simulink model "unicycle"  (R2025b)
settings: Solver=ode5  StartTime=0.0  StopTime=40  FixedStep=1e-3  MaxStep=0.01  RelTol=1e-3
libraries: dspsigops x1
settings Model: Creator=Cris  LastModifiedBy=Cris
settings DebuggingCC: UnderspecifiedInitializationDetection=Classic  MergeDetectMultiDrivingBlocksExec=none
settings ModelReferenceCC: PropagateSignalLabelsOutOfModel=off

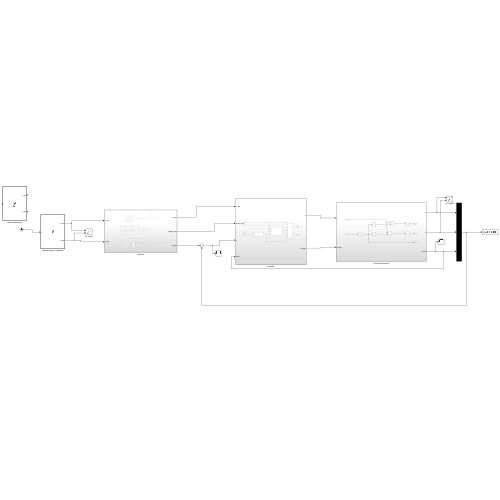
[thumbnail: Simulink's stored preview of the top-level diagram]
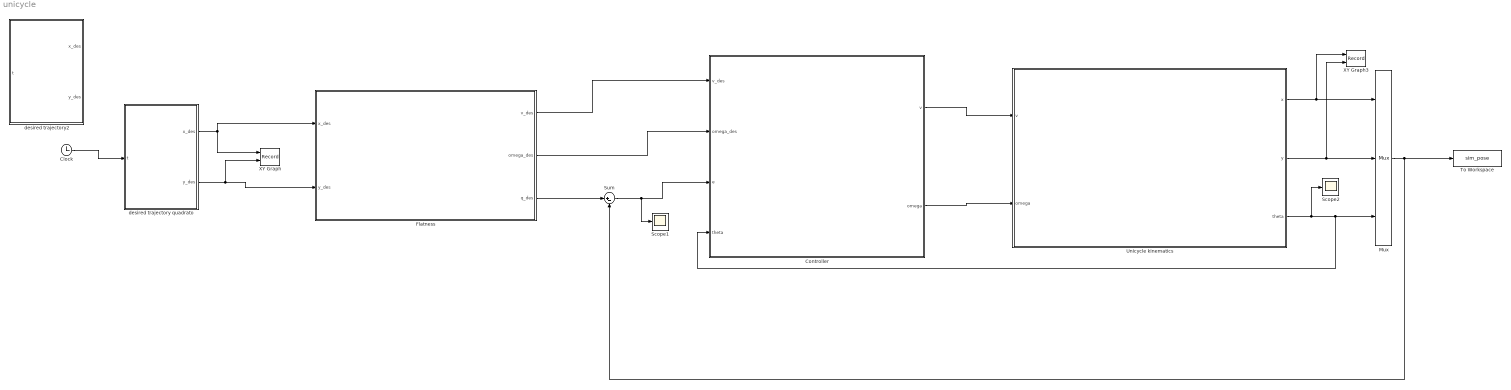
== system unicycle ==
  Clock : Clock
  Controller : Subsystem
  Flatness : Subsystem
  Mux : Mux  Inputs=3
  Scope1 : Scope
      settings: ActiveDisplayYMinimum=-1  ActiveDisplayYMaximum=1  DataLoggingVariableName=ScopeData3  DataLoggingSaveFormat=Array
  Scope2 : Scope
      settings: ActiveDisplayYMinimum=-1.1717356950439886  ActiveDisplayYMaximum=10.422944252013369  DataLoggingSaveFormat=Array
  Sum : Sum  Inputs=|+-
  To Workspace : ToWorkspace  VariableName=sim_pose  SaveFormat=Timeseries  SampleTime=-1
  Unicycle kinematics : Subsystem
  XY Graph : Record  NumPorts=2.0  FileSettingsInternal="{\"entries\":[{\"content\":{\"excelSettings\":{\"content\":{},\"type\":\"Streamout.ExcelSettings\"},\"parquetSettings\":{\"content\":{},\"type\":\"Streamout.ParquetSettings\"}},\"type\":\"Streamout.FileSettingStorage\",\"uuid\":\"\"}],\"packageUris\":[\"http:\\/\\/schema.mathworks.com\\/mf0\\/streamout_blocks\\/R2020a\"],\"version\":\"1.0\"}"  FrameSettings=[0, 0]  Layout=[1 1]  SignalsInternal="{\"entries\":[{\"content\":{\"signals\":[{\"content\":{\"blockPath\":[],\"dimensions\":[1],\"domain\":\"\",\"lineColor\":\"#a2142f\",\"plots\":[ 1 ],\"port\":1,\"sid\":[\"\"],\"signalID\":1,\"signalName\":\"desired trajectory quadrato:1\"},\"type\":\"RecordBlkView.Signal\",\"uuid\":\"\"},{\"content\":{\"blockPath\":[],\"dimensions\":[1],\"domain\":\"\",\"lineColor\":\"#139fff\",\"plots\":[ 1 ],\"port\":2,\"sid\":[\"\"],\"signalID\":2,\"signalName\":\"desired trajectory quadrato:2\"},\"type\":\"RecordBlkView.Signal\",\"uuid\":\"\"}]},\"type\":\"RecordBlkView.InputSignals\",\"uuid\":\"\"}],\"packageUris\":[\"http:\\/\\/schema.mathworks.com\\/mf0\\/streamout_blocks\\/R2020a\"],\"version\":\"1.0\"}"  VisualizationBindings="{\"xyplotplugin\":{\"info\":[{\"series\":[{\"bindingParametersList\":[{\"parameter\":\"X-Axis\",\"signalID\":1,\"signalName\":\"desired trajectory quadrato:1\"},{\"parameter\":\"Y-Axis\",\"signalID\":2,\"signalName\":\"desired trajectory quadrato:2\"}],\"seriesID\":0}],\"subplotID\":1}]}}"  CompatibilityTag=XY
  XY Graph3 : Record  NumPorts=2.0  FileSettingsInternal="{\"entries\":[{\"content\":{\"excelSettings\":{\"content\":{},\"type\":\"Streamout.ExcelSettings\"},\"parquetSettings\":{\"content\":{},\"type\":\"Streamout.ParquetSettings\"}},\"type\":\"Streamout.FileSettingStorage\",\"uuid\":\"\"}],\"packageUris\":[\"http:\\/\\/schema.mathworks.com\\/mf0\\/streamout_blocks\\/R2020a\"],\"version\":\"1.0\"}"  FrameSettings=[0, 0]  Layout=[1 1]  SignalsInternal="{\"entries\":[{\"content\":{\"signals\":[{\"content\":{\"blockPath\":[],\"dimensions\":[1],\"domain\":\"\",\"lineColor\":\"#a2142f\",\"plots\":[ 1 ],\"port\":1,\"sid\":[\"\"],\"signalID\":1,\"signalName\":\"Unicycle kinematics:1\"},\"type\":\"RecordBlkView.Signal\",\"uuid\":\"\"},{\"content\":{\"blockPath\":[],\"dimensions\":[1],\"domain\":\"\",\"lineColor\":\"#139fff\",\"plots\":[ 1 ],\"port\":2,\"sid\":[\"\"],\"signalID\":2,\"signalName\":\"Unicycle kinematics:2\"},\"type\":\"RecordBlkView.Signal\",\"uuid\":\"\"}]},\"type\":\"RecordBlkView.InputSignals\",\"uuid\":\"\"}],\"packageUris\":[\"http:\\/\\/schema.mathworks.com\\/mf0\\/streamout_blocks\\/R2020a\"],\"version\":\"1.0\"}"  VisualizationBindings="{\"xyplotplugin\":{\"info\":[{\"series\":[{\"bindingParametersList\":[{\"parameter\":\"X-Axis\",\"signalID\":1,\"signalName\":\"Unicycle kinematics:1\"},{\"parameter\":\"Y-Axis\",\"signalID\":2,\"signalName\":\"Unicycle kinematics:2\"}],\"seriesID\":0}],\"subplotID\":1}]}}"  CompatibilityTag=XY
  desired trajectory quadrato : MATLAB Function  TreatAsAtomicUnit=on
  desired trajectory2 : MATLAB Function  TreatAsAtomicUnit=on
  wires:
  Flatness/1(v_des) -> Controller/1(v_des)
  Flatness/2(omega_des) -> Controller/2(omega_des)
  Flatness/3(q_des) -> Sum/1
  Sum/1 -> Scope1/1, Controller/3(e)
  Unicycle kinematics/1(x) -> XY Graph3/1, Mux/1
  Unicycle kinematics/2(y) -> XY Graph3/2, Mux/2
  Unicycle kinematics/3(theta) -> Scope2/1, Controller/4(theta), Mux/3
  Mux/1 -> To Workspace/1, Sum/2
  Controller/2(omega) -> Unicycle kinematics/2(omega)
  Controller/1(v) -> Unicycle kinematics/1(v)
  desired trajectory quadrato/1(x_des) -> Flatness/1(x_des), XY Graph/1
  desired trajectory quadrato/2(y_des) -> Flatness/2(y_des), XY Graph/2
  Clock/1 -> desired trajectory quadrato/1(t)

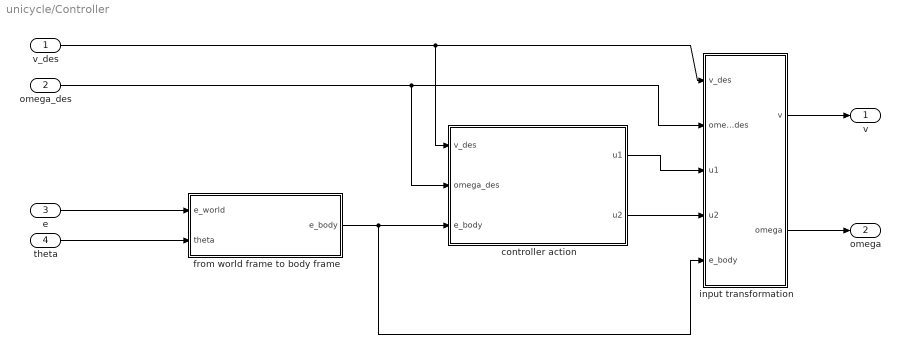
== system unicycle/Controller ==
  v_des : Inport
  omega_des : Inport  Port=2
  e : Inport  Port=3
  theta : Inport  Port=4
  controller action : MATLAB Function  TreatAsAtomicUnit=on
  from world frame to body frame : MATLAB Function  TreatAsAtomicUnit=on
  input transformation : MATLAB Function  TreatAsAtomicUnit=on
  v : Outport
  omega : Outport  Port=2
  wires:
  e/1 -> from world frame to body frame/1(e_world)
  theta/1 -> from world frame to body frame/2(theta)
  from world frame to body frame/1(e_body) -> input transformation/5(e_body), controller action/3(e_body)
  v_des/1 -> controller action/1(v_des), input transformation/1(v_des)
  controller action/2(u2) -> input transformation/4(u2)
  input transformation/2(omega) -> omega/1
  input transformation/1(v) -> v/1
  omega_des/1 -> input transformation/2(omega_des), controller action/2(omega_des)
  controller action/1(u1) -> input transformation/3(u1)

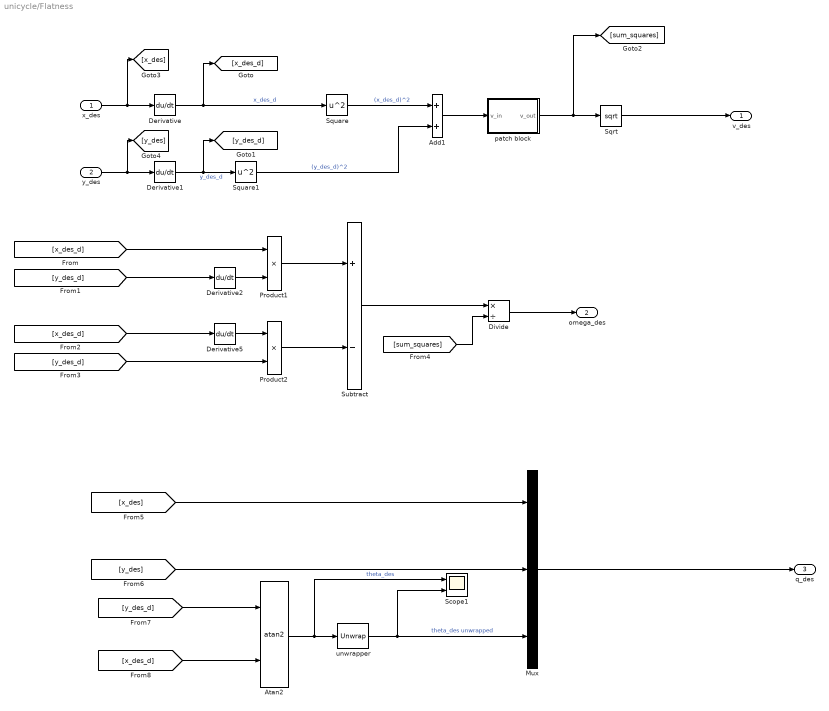
== system unicycle/Flatness ==
  x_des : Inport
  y_des : Inport  Port=2
  Add1 : Sum
  Atan2 : Trigonometry  Operator=atan2
  Derivative{,1..2,5} (4 alike) : Derivative
  Divide : Product  Inputs=*/
  Mux : Mux  Inputs=3
  Product1 : Product
  Product2 : Product
  Scope1 : Scope  NumInputPorts=2
      settings: ActiveDisplayYMinimum=-2.3561944901923448  ActiveDisplayYMaximum=5.497787143782138  DataLoggingVariableName=ScopeData2  DataLoggingSaveFormat=Array
  Sqrt : Sqrt
  Square : Math  Operator=square
  Square1 : Math  Operator=square
  Subtract : Sum  Inputs=+-
  patch block : MATLAB Function  TreatAsAtomicUnit=on
  unwrapper : dspsigops/Unwrap  tol=pi  InputProcessing=Columns as channels (frame based)  running=off
  v_des : Outport
  omega_des : Outport  Port=2
  q_des : Outport  Port=3
  wires:
  x_des/1 -> [x_des], Derivative/1
  y_des/1 -> [y_des], Derivative1/1
  Derivative/1 -> [x_des_d], Square/1  "x_des_d"
  Derivative1/1 -> [y_des_d], Square1/1  "y_des_d"
  Square/1 -> Add1/1  "(x_des_d)^2"
  Square1/1 -> Add1/2  "(y_des_d)^2"
  [x_des_d] -> Product1/1
  [y_des_d] -> Derivative2/1
  Derivative2/1 -> Product1/2
  [y_des_d] -> Product2/2
  [x_des_d] -> Derivative5/1
  Derivative5/1 -> Product2/1
  Product1/1 -> Subtract/1
  Product2/1 -> Subtract/2
  Subtract/1 -> Divide/1
  [sum_squares] -> Divide/2
  Divide/1 -> omega_des/1
  Mux/1 -> q_des/1
  Atan2/1 -> unwrapper/1, Scope1/1  "theta_des"
  [x_des_d] -> Atan2/2
  [y_des_d] -> Atan2/1
  Add1/1 -> patch block/1(v_in)
  patch block/1(v_out) -> [sum_squares], Sqrt/1
  Sqrt/1 -> v_des/1
  [x_des] -> Mux/1
  [y_des] -> Mux/2
  unwrapper/1 -> Mux/3, Scope1/2  "theta_des unwrapped"

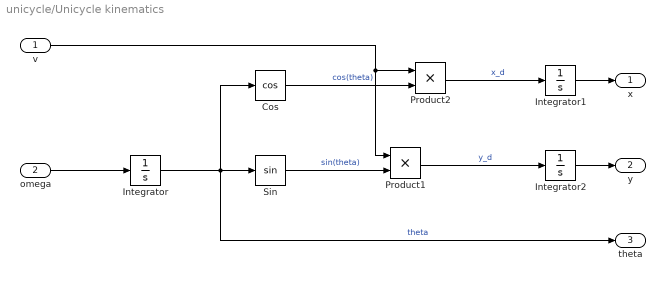
== system unicycle/Unicycle kinematics ==
  v : Inport
  omega : Inport  Port=2
  Cos : Trigonometry  Operator=cos
  Integrator : Integrator
  Integrator1 : Integrator
  Integrator2 : Integrator
  Product1 : Product
  Product2 : Product
  Sin : Trigonometry
  x : Outport
  y : Outport  Port=2
  theta : Outport  Port=3
  wires:
  omega/1 -> Integrator/1
  Integrator/1 -> theta/1, Cos/1, Sin/1  "theta"
  Cos/1 -> Product2/2  "cos(theta)"
  Sin/1 -> Product1/2  "sin(theta)"
  v/1 -> Product2/1, Product1/1
  Integrator1/1 -> x/1
  Product2/1 -> Integrator1/1  "x_d"
  Integrator2/1 -> y/1
  Product1/1 -> Integrator2/1  "y_d"

== matlab function unicycle/Controller/controller action ==
  data: v_des input; omega_des input; e_body input; u1 output; u2 output
function [u1, u2] = fcn(v_des, omega_des, e_body)

% TO DO: parametri da modfiicare
d = 1/sqrt(2);
a = 10;



% parametri controllore
k1 = 2*d*a;

% if abs(v_des) < 1e-4
%     if v_des >= 0
%         v_des = 1e-4;
%     else
%         v_des = -1e-4;
%     end
% end

k3 = k1;
k2 = ( a^2-(omega_des)^2 ) / v_des;

u1 = [-k1, 0, 0] * e_body;
u2 = [0, -k2, -k3] * e_body;

== matlab function unicycle/Controller/from world frame to body frame ==
  data: e_world input; e_body output size=3; theta input
function e_body = fcn(e_world, theta)


% Transformation matrix
R = [cos(theta), sin(theta), 0; 
    -sin(theta), cos(theta), 0;
    0, 0, 1];

% get error in body frame
e_body = R*e_world;

== matlab function unicycle/Controller/input transformation ==
  data: v_des input; v output size=1; omega_des input; u1 input; u2 input; e_body input size=3; omega output
function [v, omega] = fcn(v_des, omega_des, u1, u2, e_body)


v = v_des * cos(e_body(3)) - u1;
omega = omega_des - u2;

== matlab function unicycle/Flatness/patch block ==
  data: v_in input size=1; v_out output size=1
function v_out = fcn(v_in)

if abs(v_in) < 1e-4
    if v_in >= 0
        v_in = 1e-4;
    else
        v_in = -1e-4;
    end
end
v_out = v_in;

== matlab function unicycle/desired trajectory quadrato ==
  data: t input; x_des output; y_des output
function [x_des, y_des] = fcn(t)

% % configurable:
% radius = 5;
% omega_des = 0.2;
% 
% % desired trajectory
% x_des = -radius*cos(omega_des*t);
% y_des = -radius*sin(omega_des*t);


% % configurable:
% radius = 10;
% omega_des = 0.5;
% 
% % desired trajectory
% x_des = radius*cos(omega_des*t);
% y_des = radius*sin(omega_des*t);
% 


if t <= 10
    x_des = 10+t;
    y_des = 10;
elseif  t <= 20
    x_des = 20;
    y_des = 0+t;
elseif  t <= 30
    x_des = 40-t;
    y_des = 20;
elseif  t <= 40
    x_des = 10;
    y_des = 50-t;
else
    x_des = 100;
    y_des = 100;
end

== matlab function unicycle/desired trajectory2 ==
  data: t input; x_des output; y_des output
function [x_des, y_des] = fcn(t)

% % configurable:
% radius = 5;
% omega_des = 0.2;
% 
% % desired trajectory
% x_des = -radius*cos(omega_des*t);
% y_des = -radius*sin(omega_des*t);


% configurable:
radius = 20;
omega_des = 5;

% desired trajectory
x_des = radius*cos(omega_des*t);
y_des = radius*sin(omega_des*t);



% if t<=10
%     x_des = 10+t;
%     y_des = 10;
% elseif  t<=20
%     x_des = 20;
%     y_des = 10+t;
% elseif  t<=30
%     x_des = 20-t;
%     y_des = 20;
% elseif  t<=40
%     x_des = 10;
%     y_des = 20-t;
% else
%     x_des = 0;
%     y_des = 0;
% end
